simulink model "Model"  (R2015a)
settings: Solver=ode45  StartTime=0.0  StopTime=10.0  RelTol=1e-3
undefined symbols (not defined in the file): magnitude
settings Model: Creator=spachaimuthu  LastModifiedBy=spachaimuthu

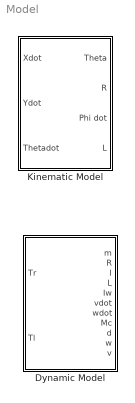
== system Model ==
  Dynamic Model : Subsystem
  Kinematic Model : Subsystem

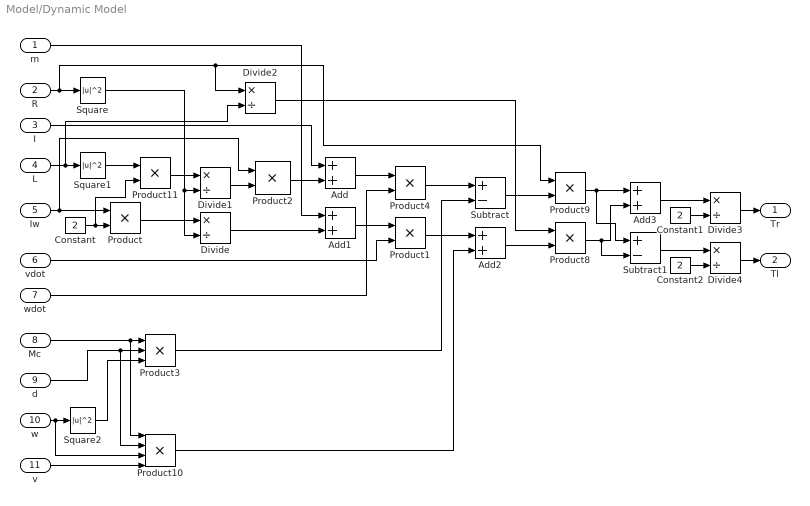
== system Model/Dynamic Model ==
  m : Inport
  R : Inport  Port=2
  I : Inport  Port=3
  L : Inport  Port=4
  Iw : Inport  Port=5
  vdot : Inport  Port=6
  wdot : Inport  Port=7
  Mc : Inport  Port=8
  d : Inport  Port=9
  w : Inport  Port=10
  v : Inport  Port=11
  Add{,1..3} (4 alike) : Sum
  Constant : Constant  Value=2
  Constant1 : Constant  Value=2
  Constant2 : Constant  Value=2
  Divide{,1..4} (5 alike) : Product  Inputs=*/
  Product{,1..2,4,8..9,11} (7 alike) : Product  RndMeth=Zero
  Product10 : Product  Inputs=4  RndMeth=Zero
  Product3 : Product  Inputs=3  RndMeth=Zero
  Square : Math  Operator=magnitude^2  SaturateOnIntegerOverflow=on
  Square1 : Math  Operator=magnitude^2  SaturateOnIntegerOverflow=on
  Square2 : Math  Operator=magnitude^2  SaturateOnIntegerOverflow=on
  Subtract : Sum  Inputs=+-
  Subtract1 : Sum  Inputs=+-
  Tr : Outport
  Tl : Outport  Port=2
  wires:
  Iw/1 -> Product2/1, Product/1
  Constant/1 -> Product11/2, Product/2
  R/1 -> Divide2/1, Product9/1, Square/1
  Product/1 -> Divide/1
  Square/1 -> Divide1/2, Divide/2
  L/1 -> Divide2/2, Square1/1
  Square1/1 -> Product11/1
  Product11/1 -> Divide1/1
  Divide1/1 -> Product2/2
  Product2/1 -> Add/2
  I/1 -> Add/1
  Divide/1 -> Add1/2
  m/1 -> Add1/1
  Add1/1 -> Product1/1
  vdot/1 -> Product1/2
  Add/1 -> Product4/1
  wdot/1 -> Product4/2
  Mc/1 -> Product10/1, Product3/1
  d/1 -> Product3/2, Product10/2
  w/1 -> Product10/3, Square2/1
  Square2/1 -> Product3/3
  v/1 -> Product10/4
  Product4/1 -> Subtract/1
  Product3/1 -> Subtract/2
  Product1/1 -> Add2/1
  Product10/1 -> Add2/2
  Subtract/1 -> Product9/2
  Add2/1 -> Product8/2
  Divide2/1 -> Product8/1
  Product9/1 -> Subtract1/1, Add3/1
  Product8/1 -> Subtract1/2, Add3/2
  Add3/1 -> Divide3/1
  Divide3/1 -> Tr/1
  Constant1/1 -> Divide3/2
  Divide4/1 -> Tl/1
  Constant2/1 -> Divide4/2
  Subtract1/1 -> Divide4/1

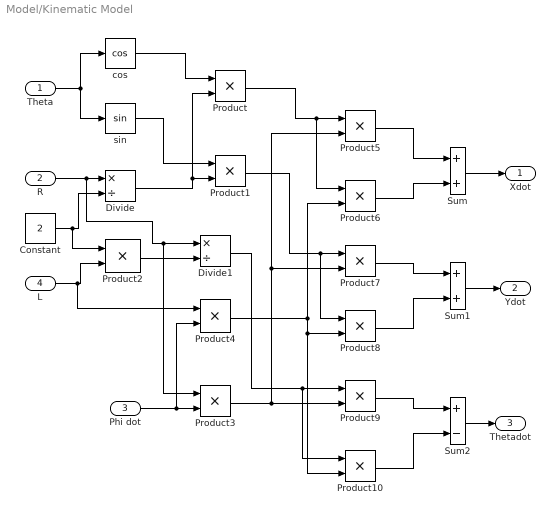
== system Model/Kinematic Model ==
  Theta : Inport
  R : Inport  Port=2
  Phi dot : Inport  Port=3
  L : Inport  Port=4
  Constant : Constant  Value=2
  Divide : Product  Inputs=*/
  Divide1 : Product  Inputs=*/
  Product{,1..10} (11 alike) : Product  RndMeth=Zero
  Sum : Sum
  Sum1 : Sum
  Sum2 : Sum  Inputs=+-
  cos : Trigonometry  Operator=cos
  sin : Trigonometry
  Xdot : Outport
  Ydot : Outport  Port=2
  Thetadot : Outport  Port=3
  wires:
  Sum/1 -> Xdot/1
  Sum1/1 -> Ydot/1
  Sum2/1 -> Thetadot/1
  Theta/1 -> cos/1, sin/1
  R/1 -> Product3/1, Divide1/1, Divide/1
  Constant/1 -> Product2/1, Divide/2
  cos/1 -> Product/1
  Divide/1 -> Product1/2, Product/2
  sin/1 -> Product1/1
  L/1 -> Product4/1, Product2/2
  Product2/1 -> Divide1/2
  Phi dot/1 -> Product4/2, Product3/2
  Product/1 -> Product6/1, Product5/1
  Product3/1 -> Product9/2, Product7/2, Product5/2
  Product4/1 -> Product10/2, Product8/2, Product6/2
  Product5/1 -> Sum/1
  Product6/1 -> Sum/2
  Product1/1 -> Product8/1, Product7/1
  Product7/1 -> Sum1/1
  Product8/1 -> Sum1/2
  Divide1/1 -> Product10/1, Product9/1
  Product9/1 -> Sum2/1
  Product10/1 -> Sum2/2
